simulink model "Roughness"  (R2021b)
settings: Solver=FixedStepDiscrete  StartTime=0.0  StopTime=300  FixedStep=0.04  RelTol=1e-3
PreLoadFcn:
  | listing = dir;
  | if (contains([listing .name], 'FLCC')) && (contains([listing .name], 'DYN'))
  |     addpath('./DYN', './FLCC', './FTG', './GPS', './INS', './MAP', './RALT');
  | elseif (contains([listing .name], 'FTG.slx'))
  |     addpath('../DYN', '../FLCC', '../FTG', '../GPS', '../INS', '../MAP', '../RALT');
  | else
  | 
  | end
  | 
  | load('BUS_STRUCTURE_DYN.mat');
  | load('BUS_STRUCTURE_FLCC.mat');
  | load('BUS_STRUCTURE_RALT.mat');
  | load('BUS_STRUCTURE_INS.mat');
  | load('BUS_STRUCTURE_GPS.mat');
  | FTG_initState;
model workspace (MAT data in the model file):
  initLLA = [0 0 0]
settings Model: ParameterArgumentNames=initLLA  Creator=ASCL  LastModifiedBy=ACUS_HVBIKE
settings SolverCC: AlgebraicLoopSolver=TrustRegion
settings DataIOCC: ExternalInput=FTGScenario.getElement('IN_Stick'),FTGScenario.getElement('IN_TF'),FTGScenario.getElement('IN_GCAS'),FTGScenario.getElement('IN_FLIGHT_CMD')  SaveOutput=off  SignalLogging=off  DSMLogging=off  SaveTime=off  ReturnWorkspaceOutputs=off
settings OptimizationCC: DefaultParameterBehavior=Inlined  UseDivisionForNetSlopeComputation=on  GainParamInheritBuiltInType=on  UseFloatMulNetSlope=on  InlineInvariantSignals=on  EnhancedBackFolding=on  PassReuseOutputArgsAs=Individual arguments  ZeroExternalMemoryAtStartup=off  ZeroInternalMemoryAtStartup=off  NoFixptDivByZeroProtection=on  EfficientFloat2IntCast=on  OptimizeBlockOrder=speed  DifferentSizesBufferReuse=on  OptimizationCustomize=off  EfficientTunableParamExpr=on
settings DebuggingCC: ParameterTunabilityLossMsg=error  SFUnexpectedBacktrackingDiag=warning  SFNoUnconditionalDefaultTransitionDiag=warning  SFMachineParentedDataDiag=warning
settings HardwareCC: ProdLongLongMode=on
settings ModelReferenceCC: ModelReferenceNumInstancesAllowed=Single
settings SFSimCC: SimUserLibraries=MAPd.lib WS2_32.LIB  MATLABDynamicMemAlloc=off
settings SFSimCC: SimCustomHeaderCode=|
  | #include "MAP.h"
  | #include "MAPDATA.h"
  | #include "DVOF.h"
  | #include "userDefined.h"
settings SFSimCC: SimUserSources=|
  | MAP.c
  | DVOF.c
  | userDefined.c
settings RTWCC: Description=Create Visual C/C++ Solution File for Embedded Coder  SystemTargetFile=ert.tlc  TemplateMakefile=RTW.MSVCBuild  GenerateReport=on  RTWUseSimCustomCode=on  CustomLibrary=MAPd.lib WS2_32.LIB  BuildConfiguration=Debug  LaunchReport=on
settings RTWCC: CustomHeaderCode=|
  | #include "MAP.h"
  | #include "MAPDATA.h"
  | #include "DVOF.h"
  | #include "userDefined.h"
settings RTWCC: CustomSource=|
  | MAP.c
  | DVOF.c
  | userDefined.c
settings CodeAppCC: ForceParamTrailComments=on  IgnoreCustomStorageClasses=off  OperatorAnnotations=on  SimulinkDataObjDesc=on  SFDataObjDesc=on  InsertBlockDesc=on  EnableCustomComments=on
settings ERTTargetCC: TargetLangStandard=C99 (ISO)  GenerateSampleERTMain=on  InlinedParameterPlacement=NonHierarchical  ERTCustomFileTemplate=example_file_process.tlc

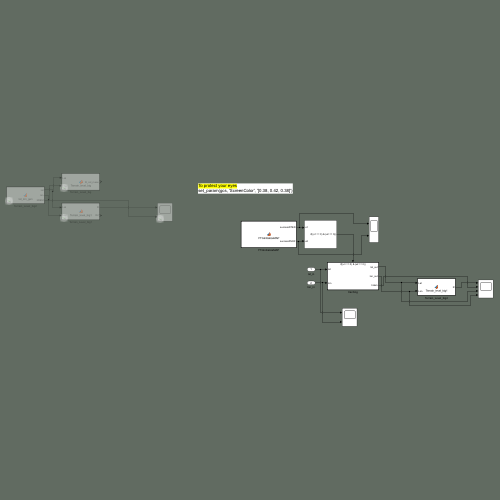
[thumbnail: Simulink's stored preview of the top-level diagram]
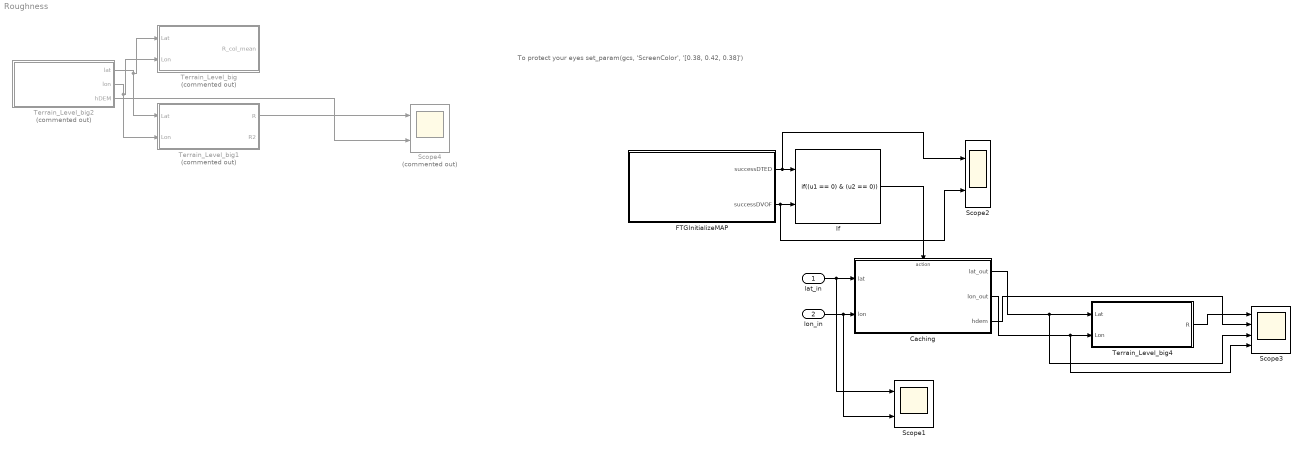
== system Roughness ==
  note: To protect your eyes
      | set_param(gcs, 'ScreenColor', '[0.38, 0.42, 0.38]')
  lat_in : Inport
  lon_in : Inport  Port=2
  Caching : Subsystem  TreatAsAtomicUnit=on
  FTGInitializeMAP : MATLAB Function  TreatAsAtomicUnit=on
  If : If  NumInputs=2  IfExpression=(u1 == 0) & (u2 == 0)  ShowElse=off
  Scope1 : Scope  NumInputPorts=2
  Scope2 : Scope  NumInputPorts=2
  Scope3 : Scope  NumInputPorts=4
  Scope4 : Scope  Commented=on  NumInputPorts=2
  Terrain_Level_big : MATLAB Function  Commented=on  TreatAsAtomicUnit=on
  Terrain_Level_big1 : MATLAB Function  Commented=on  TreatAsAtomicUnit=on
  Terrain_Level_big2 : MATLAB Function  Commented=on  TreatAsAtomicUnit=on
  Terrain_Level_big4 : MATLAB Function  TreatAsAtomicUnit=on
  wires:
  Terrain_Level_big1/1(R) -> Scope4/1
  Terrain_Level_big2/1(lat) -> Terrain_Level_big1/1(Lat), Terrain_Level_big/1(Lat)
  Terrain_Level_big2/2(lon) -> Terrain_Level_big1/2(Lon), Terrain_Level_big/2(Lon)
  Terrain_Level_big2/3(hDEM) -> Scope4/2
  If/1 -> Caching/Action
  FTGInitializeMAP/2(successDVOF) -> Scope2/2, If/2
  FTGInitializeMAP/1(successDTED) -> Scope2/1, If/1
  Caching/1(lat_out) -> Scope3/3, Terrain_Level_big4/1(Lat)
  Caching/2(lon_out) -> Scope3/4, Terrain_Level_big4/2(Lon)
  Caching/3(hdem) -> Scope3/2
  Terrain_Level_big4/1(R) -> Scope3/1
  lat_in/1 -> Scope1/1, Caching/1(lat)
  lon_in/1 -> Scope1/2, Caching/2(lon)

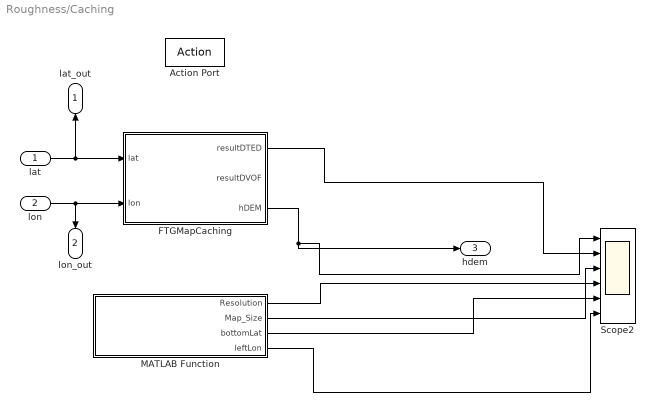
== system Roughness/Caching ==
  lat : Inport
  lon : Inport  Port=2
  Action Port : ActionPort  ActionPortLabel=if((u1 == 0) & (u2 == 0))
  FTGMapCaching : MATLAB Function  TreatAsAtomicUnit=on
  MATLAB Function : MATLAB Function  TreatAsAtomicUnit=on
  Scope2 : Scope  NumInputPorts=6
  lat_out : Outport
  lon_out : Outport  Port=2
  hdem : Outport  Port=3
  wires:
  lat/1 -> FTGMapCaching/1(lat), lat_out/1
  lon/1 -> FTGMapCaching/2(lon), lon_out/1
  MATLAB Function/3(bottomLat) -> Scope2/5
  MATLAB Function/1(Resolution) -> Scope2/4
  MATLAB Function/4(leftLon) -> Scope2/6
  FTGMapCaching/3(hDEM) -> hdem/1, Scope2/1
  MATLAB Function/2(Map_Size) -> Scope2/3
  FTGMapCaching/1(resultDTED) -> Scope2/2

== matlab function Roughness/Terrain_Level_big2 ==
  data: lat output; lon output; hDEM output
function [lat, lon, hDEM] = lat_lon_gen()

lat = 35.320600;
lon = 127.701200;
hDEM = double(0.0);

hDEM = coder.ceval('GetElevation', lat, lon);

end

== matlab function Roughness/Caching/MATLAB Function ==
  data: Resolution output; Map_Size output; bottomLat output; leftLon output
function [Resolution, Map_Size, bottomLat, leftLon] = ReturnBottomLeftLatLon

Resolution = double(0.0);
Map_Size = double(0.0);

leftLon = 0.0;
leftLon = coder.ceval('ReturnLeftLon');

bottomLat = 0.0;
bottomLat = coder.ceval('ReturnBottomLat');

end

== matlab function Roughness/Terrain_Level_big4 ==
  data: Lat input; Lon input; R output
function R = Terrain_level_big1(Lat, Lon)

R=Terrain_level(Lat, Lon);

end

== matlab function Roughness/Terrain_Level_big ==
  data: Lat input; Lon input; R_col_mean output
function R_col_mean = Terrain_level_big(Lat, Lon)

% value init
lat2m = 110961.7060516;
lon2m = 89476.51124;
Init_value = zeros(2,9999);
d_Lat = 90/lat2m; d_Lon = 90/lon2m;
size = 5;                                                        % 5x5 분
length_lat_min = round((size/60*lat2m)/180);                     % 프로파일 크기 180x180m
length_lon_min = round((size/60*lon2m)/180);                     % 프로파일 크기 180x180m

R_col = zeros(length_lat_min, length_lon_min);

% Init lat, lon Calculate
Init_value(1) = Lat + (d_Lat*2)*((length_lat_min-1)/2);
Init_value(2) = Lon - (d_Lon*2)*((length_lon_min-1)/2);

% n*n roughtness calculate
for i = 1 : 1 : length_lat_min
    for j = 1 : 1 : length_lon_min
        % Call "Terrain_level" fcn
        Lat_i = Init_value(1) - (i-1)*(d_Lat*2);
        Lon_i = Init_value(2) + (j-1)*(d_Lon*2);
        R_col(i, j) = Terrain_level(Lat_i, Lon_i);
    end
end

% roughtness mean calculate
R_col_mean = mean(mean(R_col));

end

== matlab function Roughness/Terrain_Level_big1 ==
  data: Lat input; Lon input; R output; R2 output
function [R,R2] = Terrain_level_big1(Lat, Lon)

% value init
lat2m = 110961.7060516;
lon2m = 89476.51124;
Init_value = zeros(2,9999);
d_Lat = 90/lat2m; d_Lon = 90/lon2m;
size = 5;                                                        % 5x5 분
length_lat_min = round((size/60*lat2m)/180);                     % 프로파일 크기 180x180m
length_lon_min = round((size/60*lon2m)/180);                     % 프로파일 크기 180x180m

SLP_CR = zeros(length_lat_min, length_lon_min);
SLP_DR = zeros(length_lat_min, length_lon_min);

% Init lat, lon Calculate
Init_value(1) = Lat + (d_Lat*2)*((length_lat_min-1)/2);
Init_value(2) = Lon - (d_Lon*2)*((length_lon_min-1)/2);

% n*n roughtness calculate
for i = 1 : 1 : length_lat_min
    for j = 1 : 1 : length_lon_min
        % Call "Terrain_level" fcn
        Lat_i = Init_value(1) - (i-1)*(d_Lat*2);                           % 초기 Lat 좌표
        Lon_i = Init_value(2) + (j-1)*(d_Lon*2);                           % 초기 Lon 좌표
        [SLP_CR(i, j), SLP_DR(i, j)] = Terrain_level2(Lat_i, Lon_i);
    end
end

% roughtness mean calculate
% R_col_mean = mean(mean(R_col));
mean_R=((mean2(SLP_CR)-mean2(SLP_DR))/2)^2;
std_R=((std(std(SLP_CR))^2)+(std(std(SLP_DR))^2))/2;
std_R2=((std(SLP_CR(:))^2)+(std(SLP_DR(:))^2))/2;

R=sqrt(mean_R+std_R)*100;
R2=sqrt(mean_R+std_R2)*100;

end

== matlab function Roughness/Caching/FTGMapCaching ==
  data: resultDTED output; resultDVOF output; lat input; lon input; hDEM output
function [resultDTED, resultDVOF, hDEM] = FTGMapCaching(lat, lon)

resultDTED = uint32(1);
resultDVOF = int32(1);
hDEM = double(0.0);                                 %%20220419

resultDVOF = coder.ceval('UpdateObstList', lat, lon);
resultDTED = coder.ceval('UpdateMapCache', lat, lon);
hDEM = coder.ceval('GetElevation', lat, lon);       %%20220419

== matlab function Roughness/FTGInitializeMAP ==
  data: successDTED output; successDVOF output
function [successDTED, successDVOF] = FTGInitializeMAP()

flagDTED = int32(1);
flagDVOF = int32(1);

pathDTED = 'C:\MAP\MAP_DB';
pathDVOF = 'C:\MAP\DVOF';

strLenDTED = int32(strlength(pathDTED));
strLenDVOF = int32(strlength(pathDVOF));

flagDTED = coder.ceval('InitialMap', pathDTED, strLenDTED );
flagDVOF = coder.ceval('InitDVOF', pathDVOF, strLenDVOF );

successDTED = flagDTED;
successDVOF = flagDVOF;
